simulink model "Decimator"  (R2023b)
settings: Solver=VariableStepAuto  StartTime=0.0  StopTime=1000/(fclk*8)  RelTol=1e-3
PreLoadFcn:
  | startup
undefined symbols (not defined in the file): fclk
libraries: hdlBasic x82, hdlsllib x2, hdlDSPIP x1, vmcUtilities x1
settings Model: Creator=andre  LastModifiedBy=andre

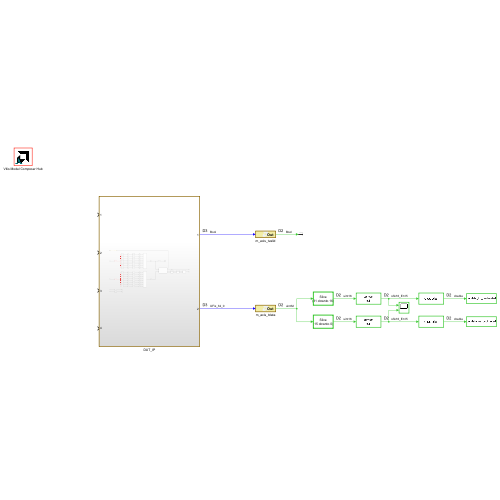
[thumbnail: Simulink's stored preview of the top-level diagram]
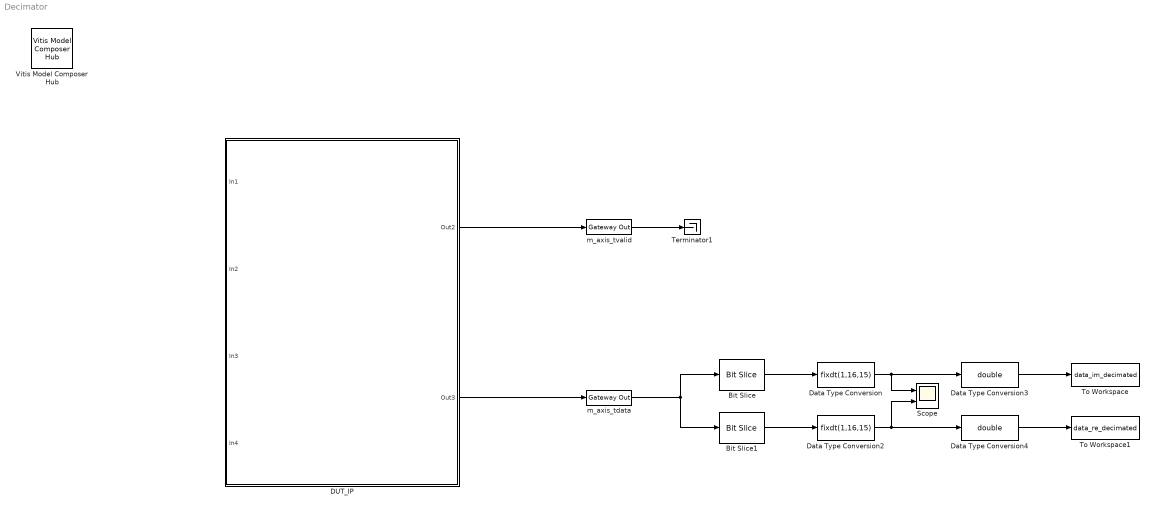
== system Decimator ==
  Bit Slice : hdlsllib/Logic and Bit Operations/Bit Slice  lidx=31  ridx=16
  Bit Slice1 : hdlsllib/Logic and Bit Operations/Bit Slice  lidx=15  ridx=0
  DUT_IP : Subsystem
  Data Type Conversion : DataTypeConversion  OutDataTypeStr=fixdt(1,16,15)  ConvertRealWorld=Stored Integer (SI)  SaturateOnIntegerOverflow=off  RndMeth=Floor
  Data Type Conversion2 : DataTypeConversion  OutDataTypeStr=fixdt(1,16,15)  ConvertRealWorld=Stored Integer (SI)  SaturateOnIntegerOverflow=off  RndMeth=Floor
  Data Type Conversion3 : DataTypeConversion  OutDataTypeStr=double  RndMeth=Floor
  Data Type Conversion4 : DataTypeConversion  OutDataTypeStr=double  RndMeth=Floor
  Scope : Scope  NumInputPorts=2
  Terminator1 : Terminator
  To Workspace : ToWorkspace  VariableName=data_im_decimated  SaveFormat=Timeseries  SampleTime=-1
  To Workspace1 : ToWorkspace  VariableName=data_re_decimated  SaveFormat=Timeseries  SampleTime=-1
  Vitis Model Composer Hub : vmcUtilities/Vitis Model Composer Hub  Tag=genX  CodeGeneration=off  SubsystemName=DUT_IP  DUTSubsystemName=DUT_IP  CompilationType=HDLCompilation  ExportTypeV2=HDL Netlist  TargetDirectory=./netlist\ip\DUT_IP\src  exportDesign=on  analyzeDesign=off  validateDesignOnHw=off  ExportType=HDL  IpVendor=xilinx.com  IpLibrary=hls  IpVersion=1.0  IpHWLanguage=Verilog  AieCompilerOptions={}  AieSimulatorOptions={}  CreateTestbench=off  TestbenchStackSize=10  RunRtlSim=off  RunCSim=off  RunAieSim=off  AieSimTimeout=50000  RunAieSimProfiling=off  LaunchVitisAnalyzer=off  PlotOutput=off  RunX86Sim=off  X86SimTimeout=10  GenHwImage=off  GenLibadfXo=on  GenHwValidationCode=off  PlatformType=Not Specified  HwSystemType=Baremetal  HwValidationTarget=hw  ProjDevice=xczu28dr-ffvg1517-2-e  ProjDevicePart=xczu28dr-ffvg1517-2-e  SamplePeriod=-1  ClockFrequency=200  DataPathParallelism=1  xilinxfamily=zynquplusRFSOC  part=xczu28dr  speed=-2-e  package=ffvg1517  directory=./netlist\ip\DUT_IP\src  testbench=off  incr_netlist=off  synthesis_tool=Vivado  clock_wrapper=Clock Enables  dbl_ovrd=According to Block Masks  dcm_input_clock_period=10  sysclk_period=(1/fclk)*(1e6)  simulink_period=1/(fclk*8)  eval_field=0  IPInfoJsonString="{\"HDLSubsystem\":{\"SubsystemName\":\"DUT_IP\",\"IPName\":\"Subsystem\",\"IPLibrary\":\"VMC\",\"IPVendor\":\"User Company\",\"IPVersion\":\"1.0\",\"TargetDirectory\":\"./netlist\",\"SubsystemDir\":\"./netlist\\\\ip\\\\DUT_IP\"},\"SubsystemTag\":\"HDLNode\"}"  LogFileName=''  NThreads=4
  m_axis_tdata : hdlBasic/Gateway Out  inherit_from_input=on  hdl_port=on  rows=1  columns=1  UseAsDAC=off  DACChannel='1'  interface=None  automatic_assignment=on  address_offset=hex2dec('00')  intf_name=''  intf_description=''  timing_constraint=None  locs_specified=off  LOCs={}  io_standard={}  XmcBlockStatus=1  maskContainerNames=group4  block_type=gatewayout  block_config=sysgen:gateway_out_config  block_width_w=590  block_height_w=620  block_width=620  block_height=750
  m_axis_tvalid : hdlBasic/Gateway Out  inherit_from_input=off  hdl_port=on  rows=1  columns=1  UseAsDAC=off  DACChannel='1'  interface=None  automatic_assignment=on  address_offset=hex2dec('00')  intf_name=''  intf_description=''  timing_constraint=None  locs_specified=off  LOCs={}  io_standard={}  XmcBlockStatus=1  maskContainerNames=group4  block_type=gatewayout  block_config=sysgen:gateway_out_config  block_width_w=590  block_height_w=620  block_width=620  block_height=750
  wires:
  m_axis_tvalid/1 -> Terminator1/1
  m_axis_tdata/1 -> Bit Slice/1, Bit Slice1/1
  Bit Slice/1 -> Data Type Conversion/1
  Bit Slice1/1 -> Data Type Conversion2/1
  Data Type Conversion/1 -> Scope/1, Data Type Conversion3/1
  Data Type Conversion2/1 -> Scope/2, Data Type Conversion4/1
  Data Type Conversion3/1 -> To Workspace/1
  Data Type Conversion4/1 -> To Workspace1/1
  DUT_IP/1(Out2) -> m_axis_tvalid/1
  DUT_IP/2(Out3) -> m_axis_tdata/1

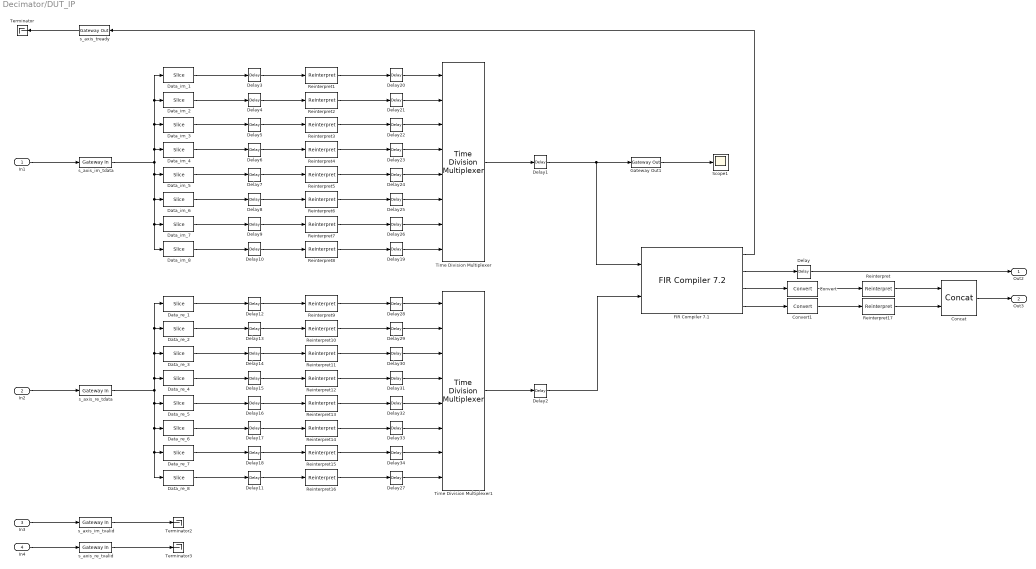
== system Decimator/DUT_IP ==
  In1 : Inport
  In2 : Inport  Port=2
  In3 : Inport  Port=3
  In4 : Inport  Port=4
  Concat : hdlBasic/Concat  num_inputs=2  XmcBlockStatus=1  maskContainerNames=group1  block_type=concat  block_config=sysgen:Concat_config
  Convert : hdlBasic/Convert  gui_display_data_type=Fixed-point  arith_type=Signed (2's comp)  n_bits=16  bin_pt=15  float_type=Single  exp_bits=8  fraction_bits=24  quantization=Truncate  overflow=Saturate  en=off  latency=1  pipeline=off  XmcBlockStatus=1  maskContainerNames=group2  block_type=convert  block_config=sysgen:Convert_config  block_width=595  block_height=885
  Convert1 : hdlBasic/Convert  gui_display_data_type=Fixed-point  arith_type=Signed (2's comp)  n_bits=16  bin_pt=15  float_type=Single  exp_bits=8  fraction_bits=24  quantization=Truncate  overflow=Saturate  en=off  latency=1  pipeline=off  XmcBlockStatus=1  maskContainerNames=group2  block_type=convert  block_config=sysgen:Convert_config  block_width=595  block_height=885
  Data_im_1 : hdlBasic/Slice  nbits=16  boolean_output=off  mode=Upper Bit Location + Width  bit1=127  base1=LSB of Input  bit0=16*8-(16*1)  base0=LSB of Input  XmcBlockStatus=1  maskContainerNames=group1  block_type=slice  block_config=sysgen:Slice_config
  Data_im_2 : hdlBasic/Slice  nbits=16  boolean_output=off  mode=Upper Bit Location + Width  bit1=111  base1=LSB of Input  bit0=16*8-(16*1)  base0=LSB of Input  XmcBlockStatus=1  maskContainerNames=group1  block_type=slice  block_config=sysgen:Slice_config
  Data_im_3 : hdlBasic/Slice  nbits=16  boolean_output=off  mode=Upper Bit Location + Width  bit1=95  base1=LSB of Input  bit0=16*8-(16*1)  base0=LSB of Input  XmcBlockStatus=1  maskContainerNames=group1  block_type=slice  block_config=sysgen:Slice_config
  Data_im_4 : hdlBasic/Slice  nbits=16  boolean_output=off  mode=Upper Bit Location + Width  bit1=79  base1=LSB of Input  bit0=16*8-(16*1)  base0=LSB of Input  XmcBlockStatus=1  maskContainerNames=group1  block_type=slice  block_config=sysgen:Slice_config
  Data_im_5 : hdlBasic/Slice  nbits=16  boolean_output=off  mode=Upper Bit Location + Width  bit1=63  base1=LSB of Input  bit0=16*8-(16*1)  base0=LSB of Input  XmcBlockStatus=1  maskContainerNames=group1  block_type=slice  block_config=sysgen:Slice_config
  Data_im_6 : hdlBasic/Slice  nbits=16  boolean_output=off  mode=Upper Bit Location + Width  bit1=47  base1=LSB of Input  bit0=16*8-(16*1)  base0=LSB of Input  XmcBlockStatus=1  maskContainerNames=group1  block_type=slice  block_config=sysgen:Slice_config
  Data_im_7 : hdlBasic/Slice  nbits=16  boolean_output=off  mode=Upper Bit Location + Width  bit1=31  base1=LSB of Input  bit0=16*8-(16*1)  base0=LSB of Input  XmcBlockStatus=1  maskContainerNames=group1  block_type=slice  block_config=sysgen:Slice_config
  Data_im_8 : hdlBasic/Slice  nbits=16  boolean_output=off  mode=Upper Bit Location + Width  bit1=15  base1=LSB of Input  bit0=16*8-(16*1)  base0=LSB of Input  XmcBlockStatus=1  maskContainerNames=group1  block_type=slice  block_config=sysgen:Slice_config
  Data_re_1 : hdlBasic/Slice  nbits=16  boolean_output=off  mode=Upper Bit Location + Width  bit1=127  base1=LSB of Input  bit0=16*8-(16*1)  base0=LSB of Input  XmcBlockStatus=1  maskContainerNames=group1  block_type=slice  block_config=sysgen:Slice_config
  Data_re_2 : hdlBasic/Slice  nbits=16  boolean_output=off  mode=Upper Bit Location + Width  bit1=111  base1=LSB of Input  bit0=16*8-(16*1)  base0=LSB of Input  XmcBlockStatus=1  maskContainerNames=group1  block_type=slice  block_config=sysgen:Slice_config
  Data_re_3 : hdlBasic/Slice  nbits=16  boolean_output=off  mode=Upper Bit Location + Width  bit1=95  base1=LSB of Input  bit0=16*8-(16*1)  base0=LSB of Input  XmcBlockStatus=1  maskContainerNames=group1  block_type=slice  block_config=sysgen:Slice_config
  Data_re_4 : hdlBasic/Slice  nbits=16  boolean_output=off  mode=Upper Bit Location + Width  bit1=79  base1=LSB of Input  bit0=16*8-(16*1)  base0=LSB of Input  XmcBlockStatus=1  maskContainerNames=group1  block_type=slice  block_config=sysgen:Slice_config
  Data_re_5 : hdlBasic/Slice  nbits=16  boolean_output=off  mode=Upper Bit Location + Width  bit1=63  base1=LSB of Input  bit0=16*8-(16*1)  base0=LSB of Input  XmcBlockStatus=1  maskContainerNames=group1  block_type=slice  block_config=sysgen:Slice_config
  Data_re_6 : hdlBasic/Slice  nbits=16  boolean_output=off  mode=Upper Bit Location + Width  bit1=47  base1=LSB of Input  bit0=16*8-(16*1)  base0=LSB of Input  XmcBlockStatus=1  maskContainerNames=group1  block_type=slice  block_config=sysgen:Slice_config
  Data_re_7 : hdlBasic/Slice  nbits=16  boolean_output=off  mode=Upper Bit Location + Width  bit1=31  base1=LSB of Input  bit0=16*8-(16*1)  base0=LSB of Input  XmcBlockStatus=1  maskContainerNames=group1  block_type=slice  block_config=sysgen:Slice_config
  Data_re_8 : hdlBasic/Slice  nbits=16  boolean_output=off  mode=Upper Bit Location + Width  bit1=15  base1=LSB of Input  bit0=16*8-(16*1)  base0=LSB of Input  XmcBlockStatus=1  maskContainerNames=group1  block_type=slice  block_config=sysgen:Slice_config
  Delay{,1..34} (35 alike) : hdlBasic/Delay  rst=off  en=off  latency=1  reg_retiming=off  XmcBlockStatus=1  maskContainerNames=group1  block_type=delay  block_config=sysgen:Delay_config
  FIR Compiler 7.1 : hdlDSPIP/FIR Compiler 7.2   coefficientvector=src.getFilters.Stage1.Numerator  coefficient_sets=1  coefficient_reload=off  filter_type=Decimation  rate_change_type=Integer  interpolation_rate=1  decimation_rate=8  zero_pack_factor=1  channel_sequence=Basic  number_channels=1  pattern_list='P4-0,P4-1,P4-2,P4-3,P4-4'  number_paths=2  ratespecification=Maximum_Possible  sampleperiod=1  hardwareoversamplingrate=1  coefficient_sign=Signed  quantization=Quantize_Only  coefficient_width=16  bestprecision=on  coefficient_fractional_bits=15  coefficient_structure=Inferred  output_rounding_mode=Full_Precision  output_width=32  filter_architecture=Systolic_Multiply_Accumulate  optimization_goal=Area  optimization_list='None'  data_buffer_type=Automatic  coefficient_buffer_type=Automatic  input_buffer_type=Automatic  output_buffer_type=Automatic  preference_for_other_storage=Automatic  multi_column_support=Automatic  columnconfig='1'  inter_column_pipe_length=4  data_has_tlast=Not_Required  m_data_has_tready=off  s_data_has_fifo=off  s_data_has_tuser=Not_Required  m_data_has_tuser=Not_Required  s_config_sync_mode=On_Vector  s_config_method=Single  num_reload_slots=1  has_aclken=off  has_aresetn=off  reset_data_vector=on  trim_axipin_name=on  simulation_type=hybrid_sim  simulation_model=sysgen:xfirv7_2_cmodel  data_path_portlist={ 's_axis_data_tdata', 'm_axis_data_tdata' }  passband_min=0.0  passband_max=0.5  stopband_min=0.5  stopband_max=1.0  filter_selection=1  gui_behaviour='Sysgen_GUI'  data_sign=Signed  data_width=16  data_fractional_bits=0  data_tuser_width=1  wrapper_available=true  ip_wrap_arbitrary_binary_point=true  ip_name=FIR Compiler  ip_version=7.2  dsptool_ready=true  ipcore_usecache=true  ipcore_useipmodelcache=true  port_translation_map={ 'aclken' => 'en', 'aresetn' => 'rst' }  run_core_at_system_period=true  ipcore_xco_need_fpga_part=true  ipcore_fpga_part=[]  XmcBlockStatus=1  maskContainerNames=tabcontainer1  block_type=fir_compiler_v7_2  block_config=sysgen:rodinimport_config  block_width=820  block_height=600
  Gateway Out1 : hdlBasic/Gateway Out  inherit_from_input=off  hdl_port=off  rows=1  columns=1  UseAsDAC=off  DACChannel='1'  interface=None  automatic_assignment=on  address_offset=hex2dec('00')  intf_name=''  intf_description=''  timing_constraint=None  locs_specified=off  LOCs={}  io_standard={}  XmcBlockStatus=1  maskContainerNames=group4  block_type=gatewayout  block_config=sysgen:gateway_out_config  block_width_w=590  block_height_w=620  block_width=620  block_height=750
  Reinterpret : hdlBasic/Reinterpret  force_arith_type=on  arith_type=Unsigned  force_bin_pt=on  bin_pt=0  XmcBlockStatus=1  maskContainerNames=group1  block_type=reinterpret  block_config=sysgen:Reinterpret_config
  Reinterpret{1..16} (16 alike) : hdlBasic/Reinterpret  force_arith_type=on  arith_type="Signed  (2's comp)"  force_bin_pt=on  bin_pt=15  XmcBlockStatus=1  maskContainerNames=group1  block_type=reinterpret  block_config=sysgen:Reinterpret_config
  Reinterpret17 : hdlBasic/Reinterpret  force_arith_type=on  arith_type=Unsigned  force_bin_pt=on  bin_pt=0  XmcBlockStatus=1  maskContainerNames=group1  block_type=reinterpret  block_config=sysgen:Reinterpret_config
  Scope1 : Scope
  Terminator : Terminator
  Terminator2 : Terminator
  Terminator3 : Terminator
  Time Division Multiplexer : hdlBasic/Time Division Multiplexer  inputs=8  vin=off  Optimization=Resource  explicit_period=off  period=1  XmcBlockStatus=1  maskContainerNames=group3  block_type=tdm  block_config=sysgen:TDM_config
  Time Division Multiplexer1 : hdlBasic/Time Division Multiplexer  inputs=8  vin=off  Optimization=Resource  explicit_period=off  period=1  XmcBlockStatus=1  maskContainerNames=group3  block_type=tdm  block_config=sysgen:TDM_config
  s_axis_im_tdata : hdlBasic/Gateway In  gui_display_data_type=Fixed-point  arith_type=Unsigned  n_bits=16*8  bin_pt=0  preci_type=Single  exp_width=8  frac_width=24  rows=1  columns=1  quantization=Truncate  overflow=Saturate  period=1/fclk  UseAsADC=off  ADCChannel='1'  interface=None  automatic_assignment=on  address_offset=hex2dec('00')  intf_name=''  intf_description=''  default_value=0  timing_constraint=None  locs_specified=off  LOCs={}  io_standard={}  inherit_from_input=off  hdl_port=on  XmcBlockStatus=1  maskContainerNames=group4  block_type=gatewayin  block_config=sysgen:gateway_in_config  block_width_w=590  block_height_w=620  block_width=640  block_height=850
  s_axis_im_tvalid : hdlBasic/Gateway In  gui_display_data_type=Boolean  arith_type=Boolean  n_bits=32  bin_pt=0  preci_type=Single  exp_width=8  frac_width=24  rows=1  columns=1  quantization="Round  (unbiased: +/- Inf)"  overflow=Saturate  period=1/fclk  UseAsADC=off  ADCChannel='1'  interface=None  automatic_assignment=on  address_offset=hex2dec('00')  intf_name=''  intf_description=''  default_value=0  timing_constraint=None  locs_specified=off  LOCs={}  io_standard={}  inherit_from_input=off  hdl_port=on  XmcBlockStatus=1  maskContainerNames=group4  block_type=gatewayin  block_config=sysgen:gateway_in_config  block_width_w=590  block_height_w=620  block_width=640  block_height=850
  s_axis_re_tdata : hdlBasic/Gateway In  gui_display_data_type=Fixed-point  arith_type=Unsigned  n_bits=16*8  bin_pt=0  preci_type=Single  exp_width=8  frac_width=24  rows=1  columns=1  quantization=Truncate  overflow=Saturate  period=1/fclk  UseAsADC=off  ADCChannel='1'  interface=None  automatic_assignment=on  address_offset=hex2dec('00')  intf_name=''  intf_description=''  default_value=0  timing_constraint=None  locs_specified=off  LOCs={}  io_standard={}  inherit_from_input=off  hdl_port=on  XmcBlockStatus=1  maskContainerNames=group4  block_type=gatewayin  block_config=sysgen:gateway_in_config  block_width_w=590  block_height_w=620  block_width=640  block_height=850
  s_axis_re_tvalid : hdlBasic/Gateway In  gui_display_data_type=Boolean  arith_type=Boolean  n_bits=32  bin_pt=0  preci_type=Single  exp_width=8  frac_width=24  rows=1  columns=1  quantization="Round  (unbiased: +/- Inf)"  overflow=Saturate  period=1/fclk  UseAsADC=off  ADCChannel='1'  interface=None  automatic_assignment=on  address_offset=hex2dec('00')  intf_name=''  intf_description=''  default_value=0  timing_constraint=None  locs_specified=off  LOCs={}  io_standard={}  inherit_from_input=off  hdl_port=on  XmcBlockStatus=1  maskContainerNames=group4  block_type=gatewayin  block_config=sysgen:gateway_in_config  block_width_w=590  block_height_w=620  block_width=640  block_height=850
  s_axis_tready : hdlBasic/Gateway Out  inherit_from_input=off  hdl_port=on  rows=1  columns=1  UseAsDAC=off  DACChannel='1'  interface=None  automatic_assignment=on  address_offset=hex2dec('00')  intf_name=''  intf_description=''  timing_constraint=None  locs_specified=off  LOCs={}  io_standard={}  XmcBlockStatus=1  maskContainerNames=group4  block_type=gatewayout  block_config=sysgen:gateway_out_config  block_width_w=590  block_height_w=620  block_width=620  block_height=750
  Out2 : Outport
  Out3 : Outport  Port=2
  wires:
  Data_im_8/1 -> Delay10/1
  Data_im_4/1 -> Delay6/1
  In2/1 -> s_axis_re_tdata/1
  In1/1 -> s_axis_im_tdata/1
  Data_im_5/1 -> Delay7/1
  Data_re_5/1 -> Delay16/1
  FIR Compiler 7.1/2 -> Delay/1
  Reinterpret16/1 -> Delay27/1
  Reinterpret13/1 -> Delay32/1
  Reinterpret12/1 -> Delay31/1
  Reinterpret14/1 -> Delay33/1
  Data_re_7/1 -> Delay18/1
  Data_im_7/1 -> Delay9/1
  FIR Compiler 7.1/3 -> Convert/1
  Reinterpret10/1 -> Delay29/1
  Reinterpret17/1 -> Concat/2
  Convert/1 -> Reinterpret/1
  Reinterpret1/1 -> Delay20/1
  Reinterpret11/1 -> Delay30/1
  Reinterpret15/1 -> Delay34/1
  FIR Compiler 7.1/1 -> s_axis_tready/1
  Reinterpret3/1 -> Delay22/1
  Reinterpret9/1 -> Delay28/1
  Reinterpret4/1 -> Delay23/1
  Data_re_6/1 -> Delay17/1
  Data_re_1/1 -> Delay12/1
  Delay/1 -> Out2/1
  Data_re_8/1 -> Delay11/1
  Data_re_4/1 -> Delay15/1
  Convert1/1 -> Reinterpret17/1
  Data_re_2/1 -> Delay13/1
  Concat/1 -> Out3/1
  Data_re_3/1 -> Delay14/1
  Reinterpret7/1 -> Delay26/1
  Data_im_2/1 -> Delay4/1
  Data_im_3/1 -> Delay5/1
  Reinterpret8/1 -> Delay19/1
  Data_im_6/1 -> Delay8/1
  Reinterpret5/1 -> Delay24/1
  FIR Compiler 7.1/4 -> Convert1/1
  Reinterpret6/1 -> Delay25/1
  Reinterpret/1 -> Concat/1
  s_axis_im_tdata/1 -> Data_im_5/1, Data_im_6/1, Data_im_7/1, Data_im_8/1, Data_im_4/1, Data_im_3/1, Data_im_1/1, Data_im_2/1
  s_axis_re_tdata/1 -> Data_re_4/1, Data_re_3/1, Data_re_2/1, Data_re_1/1, Data_re_5/1, Data_re_6/1, Data_re_8/1, Data_re_7/1
  s_axis_re_tvalid/1 -> Terminator3/1
  s_axis_im_tvalid/1 -> Terminator2/1
  In3/1 -> s_axis_im_tvalid/1
  In4/1 -> s_axis_re_tvalid/1
  s_axis_tready/1 -> Terminator/1
  Gateway Out1/1 -> Scope1/1
  Time Division Multiplexer/1 -> Delay1/1
  Data_im_1/1 -> Delay3/1
  Reinterpret2/1 -> Delay21/1
  Delay1/1 -> Gateway Out1/1, FIR Compiler 7.1/1
  Time Division Multiplexer1/1 -> Delay2/1
  Delay2/1 -> FIR Compiler 7.1/2
  Delay3/1 -> Reinterpret1/1
  Delay4/1 -> Reinterpret2/1
  Delay5/1 -> Reinterpret3/1
  Delay6/1 -> Reinterpret4/1
  Delay8/1 -> Reinterpret6/1
  Delay9/1 -> Reinterpret7/1
  Delay10/1 -> Reinterpret8/1
  Delay7/1 -> Reinterpret5/1
  Delay12/1 -> Reinterpret9/1
  Delay14/1 -> Reinterpret11/1
  Delay11/1 -> Reinterpret16/1
  Delay17/1 -> Reinterpret14/1
  Delay18/1 -> Reinterpret15/1
  Delay15/1 -> Reinterpret12/1
  Delay13/1 -> Reinterpret10/1
  Delay16/1 -> Reinterpret13/1
  Delay20/1 -> Time Division Multiplexer/1
  Delay26/1 -> Time Division Multiplexer/7
  Delay21/1 -> Time Division Multiplexer/2
  Delay19/1 -> Time Division Multiplexer/8
  Delay25/1 -> Time Division Multiplexer/6
  Delay22/1 -> Time Division Multiplexer/3
  Delay23/1 -> Time Division Multiplexer/4
  Delay24/1 -> Time Division Multiplexer/5
  Delay34/1 -> Time Division Multiplexer1/7
  Delay33/1 -> Time Division Multiplexer1/6
  Delay31/1 -> Time Division Multiplexer1/4
  Delay30/1 -> Time Division Multiplexer1/3
  Delay28/1 -> Time Division Multiplexer1/1
  Delay29/1 -> Time Division Multiplexer1/2
  Delay32/1 -> Time Division Multiplexer1/5
  Delay27/1 -> Time Division Multiplexer1/8
